simulink model "Aug_MPC_UnCon"  (R2021a)
settings: Solver=FixedStepDiscrete  StartTime=0.0  StopTime=10.0  FixedStep=h  RelTol=1e-3
values from neighbouring files (symbols this model uses):
  C = sys.C    [Initialize_MPC.m]    (also in Initialize_MPC_non.m; Values_Rev3.mat = [1 0 0 0 1 0 0 0 1 0 0 0 ... (18 elements, 3x6)])
  h = 0.01    [Main_Funwork4.m]
  K_Uncons = (matrices.R + matrices.Z'*matrices.Q*matrices.Z)^-1*matrices.Z'*matrices.Q    [Main_Funwork4.m]
  m = 3    [Main_Funwork4.m]
  Np = 43    [Main_Funwork4.m]
  r_p = zeros(m*Np,1)    [Initialize_MPC.m]    (also in Initialize_MPC_non.m = zeros(3*Np,1))
undefined symbols (not defined in the file or in its folder): constraints, DiscIntNeverNeededParam, int, matrices, x0
libraries: vrlib x2, simulink x1, aerolibanimutils x1, dspvision x1
settings Model: Creator=vicen  LastModifiedBy=vicen

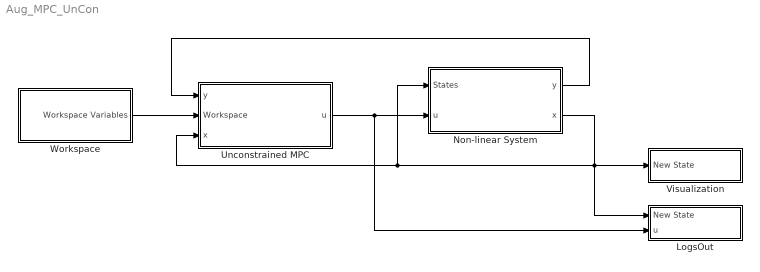
== system Aug_MPC_UnCon ==
  LogsOut : Subsystem
  Non-linear System : Subsystem
  Unconstrained MPC : Subsystem
  Visualization : Subsystem
  Workspace : Subsystem
  wires:
  Unconstrained MPC/1(u) -> LogsOut/2(u), Non-linear System/2(u)
  Non-linear System/1(y) -> Unconstrained MPC/1(y)
  Workspace/1(Workspace Variables) -> Unconstrained MPC/2(Workspace)
  Non-linear System/2(x) -> Visualization/1(New State), LogsOut/1(New State), Non-linear System/1(States), Unconstrained MPC/3(x)

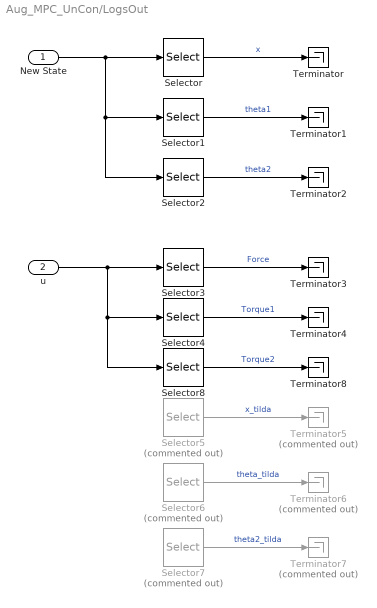
== system Aug_MPC_UnCon/LogsOut ==
  New State : Inport
  u : Inport  Port=2
  Selector : Selector  InputPortWidth=6  IndexOptions=Index vector (dialog)  Indices=1  OutputSizes=1
  Selector1 : Selector  InputPortWidth=6  IndexOptions=Index vector (dialog)  Indices=2  OutputSizes=1
  Selector2 : Selector  InputPortWidth=6  IndexOptions=Index vector (dialog)  Indices=3  OutputSizes=1
  Selector3 : Selector  InputPortWidth=3  IndexOptions=Index vector (dialog)  Indices=1  OutputSizes=1
  Selector4 : Selector  InputPortWidth=3  IndexOptions=Index vector (dialog)  Indices=2  OutputSizes=1
  Selector5 : Selector  Commented=on  InputPortWidth=6  IndexOptions=Index vector (dialog)  Indices=1  OutputSizes=1
  Selector6 : Selector  Commented=on  InputPortWidth=6  IndexOptions=Index vector (dialog)  Indices=2  OutputSizes=1
  Selector7 : Selector  Commented=on  InputPortWidth=6  IndexOptions=Index vector (dialog)  Indices=3  OutputSizes=1
  Selector8 : Selector  InputPortWidth=3  IndexOptions=Index vector (dialog)  Indices=3  OutputSizes=1
  Terminator{,1..4,8} (6 alike) : Terminator
  Terminator5 : Terminator  Commented=on
  Terminator6 : Terminator  Commented=on
  Terminator7 : Terminator  Commented=on
  wires:
  Selector/1 -> Terminator/1  "x"
  Selector1/1 -> Terminator1/1  "theta1"
  Selector2/1 -> Terminator2/1  "theta2"
  New State/1 -> Selector2/1, Selector1/1, Selector/1
  u/1 -> Selector8/1, Selector4/1, Selector3/1
  Selector4/1 -> Terminator4/1  "Torque1"
  Selector3/1 -> Terminator3/1  "Force"
  Selector5/1 -> Terminator5/1  "x_tilda"
  Selector6/1 -> Terminator6/1  "theta_tilda"
  Selector7/1 -> Terminator7/1  "theta2_tilda"
  Selector8/1 -> Terminator8/1  "Torque2"

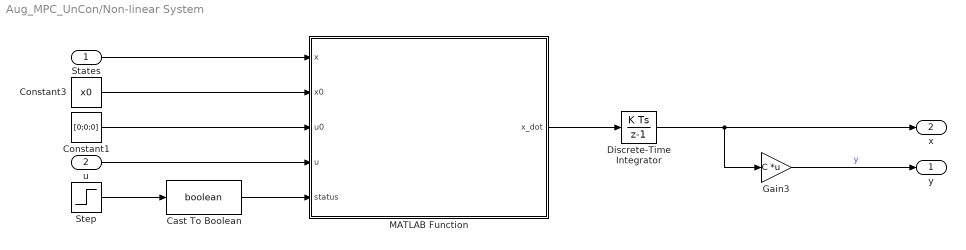
== system Aug_MPC_UnCon/Non-linear System ==
  States : Inport
  u : Inport  Port=2
  Cast To Boolean : DataTypeConversion  OutDataTypeStr=boolean
  Constant1 : Constant  Value=[0;0;0]  VectorParams1D=off
  Constant3 : Constant  Value=x0  VectorParams1D=off  OutDataTypeStr=Bus: State_bus
  Discrete-Time Integrator : DiscreteIntegrator  InitialCondition=[x0.x;x0.theta1;x0.theta2;x0.x_dot;x0.theta1_dot;x0.theta2_dot]  SampleTime=h  ICPrevOutput=DiscIntNeverNeededParam  ICPrevScaledInput=DiscIntNeverNeededParam
  Gain3 : Gain  Gain=C  Multiplication=Matrix(K*u)
  MATLAB Function : MATLAB Function  TreatAsAtomicUnit=on
  Step : Step  Time=h  SampleTime=0
  y : Outport
  x : Outport  Port=2
  wires:
  States/1 -> MATLAB Function/1(x)
  u/1 -> MATLAB Function/4(u)
  Step/1 -> Cast To Boolean/1
  Cast To Boolean/1 -> MATLAB Function/5(status)
  Gain3/1 -> y/1  "y"
  Discrete-Time Integrator/1 -> Gain3/1, x/1
  Constant3/1 -> MATLAB Function/2(x0)
  MATLAB Function/1(x_dot) -> Discrete-Time Integrator/1
  Constant1/1 -> MATLAB Function/3(u0)

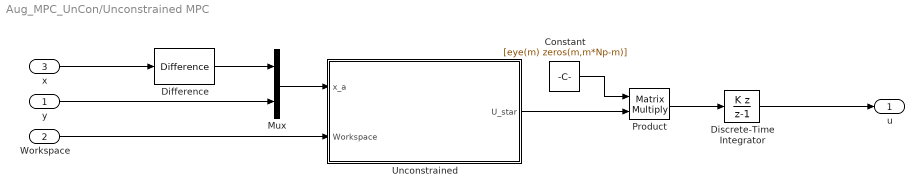
== system Aug_MPC_UnCon/Unconstrained MPC ==
  y : Inport
  Workspace : Inport  Port=2
  x : Inport  Port=3
  Constant : Constant  Value=[eye(m) zeros(m,m*Np-m)]  VectorParams1D=off
  Difference : simulink/Discrete/Difference  ICPrevInput=[x0.x;x0.theta1;x0.theta2;x0.x_dot;x0.theta1_dot;x0.theta2_dot]  OutMin=[]  OutMax=[]  OutDataType=fixdt(1, 16)  OutScaling=2^-10  DoSatur=off
  Discrete-Time Integrator : DiscreteIntegrator  IntegratorMethod=Accumulation: Backward Euler  InitialCondition=[0;0;0]  SampleTime=-1  ICPrevOutput=DiscIntNeverNeededParam  ICPrevScaledInput=DiscIntNeverNeededParam
  Mux : Mux  Inputs=2
  Product : Product  Multiplication=Matrix(*)
  Unconstrained : Subsystem
  u : Outport
  wires:
  Difference/1 -> Mux/1
  y/1 -> Mux/2
  Mux/1 -> Unconstrained/1(x_a)
  Workspace/1 -> Unconstrained/2(Workspace)
  Constant/1 -> Product/1
  Unconstrained/1(U_star) -> Product/2
  x/1 -> Difference/1
  Discrete-Time Integrator/1 -> u/1
  Product/1 -> Discrete-Time Integrator/1

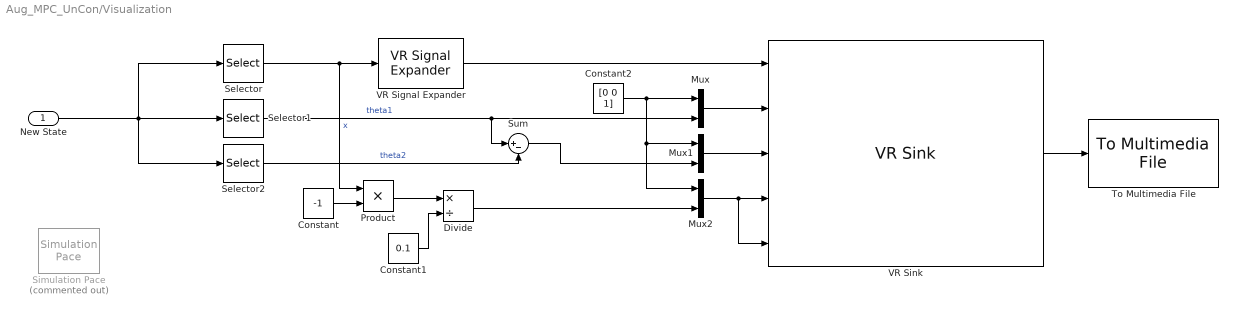
== system Aug_MPC_UnCon/Visualization ==
  New State : Inport
  Constant : Constant  Value=-1
  Constant1 : Constant  Value=0.1
  Constant2 : Constant  Value=[0 0 1]
  Divide : Product  Inputs=*/
  Mux : Mux  Inputs=2
  Mux1 : Mux  Inputs=2
  Mux2 : Mux  Inputs=2
  Product : Product
  Selector : Selector  InputPortWidth=6  IndexOptions=Index vector (dialog)  Indices=1  OutputSizes=1
  Selector1 : Selector  InputPortWidth=6  IndexOptions=Index vector (dialog)  Indices=2  OutputSizes=1
  Selector2 : Selector  InputPortWidth=6  IndexOptions=Index vector (dialog)  Indices=3  OutputSizes=1
  Simulation Pace : aerolibanimutils/Simulation Pace  Commented=on  SimulationPace=1  SleepMode=Auto  OutputPaceError=off  SampleTime=1/30
  Sum : Sum  Inputs=|+-
  To Multimedia File : dspvision/To Multimedia File  outputFilename=prob2.avi  streamSelection=Video only  videoCompressor=None (uncompressed)  audioCompressor=None (uncompressed)  imagePorts=One multidimensional signal  fileType=AVI  audioDatatype=Determine from input data type  fourcc=RGB  videoQuality=75  mj2000CompFactor=10
  VR Signal Expander : vrlib/VR Signal Expander  outwidth=3  outidx=[1]
  VR Sink : vrlib/VR Sink  InstantiateOnLoad=on  SampleTime=0.1  ViewEnable=on  RemoteChange=off  RemoteView=off  FieldsWritten=Cart.translation.3.1.1.double#Rotation1.rotation.4.1.1.double#Rotation2.rotation.4.1.1.double#Axis_Rotate.rotation.4.1.1.double#Axis_Rotate2.rotation.4.1.1.double  WorldFileName=Cart_Actual.WRL  AutoView=off  VideoDimensions=[1500 2000]  AllowVariableSize=off  FigureProperties="{'Position', 'Name', 'Viewpoint', 'CameraBound', 'CameraDirection', 'CameraPosition', 'CameraUpVector', 'ZoomFactor', 'Antialiasing', 'Headlight', 'Lighting', 'NavPanel', 'Sound', 'StatusBar', 'Stereo3D', 'Stereo3DCameraOffset', 'Stereo3DHIT', 'ToolBar', 'Textures', 'Transparency', 'Triad', 'Wireframe', 'NavZones', 'NavMode', 'NavSpeed', 'CaptureFileFormat', 'CaptureFileName', 'Record2DCompressMethod', 'Record2DCompressQuality', 'Record2D', 'Record2DFileName', 'Record2DFPS'; [1.2660000000000001e+02   9.4799999999999955e+01   8.0000000000000000e+02   6.0020000000000005e+02], '', '_untitled_1', 'on', [0.0000000000000000e+00   0.0000000000000000e+00  -1.0000000000000000e+00], [0.0000000000000000e+00   0.0000000000000000e+00   0.0000000000000000e+00], [0.0000000000000000e+00   1.0000000000000000e+00   0.0000000000000000e+00], [1.0000000000000000e+00], 'on', 'on', 'on', 'none', 'on', 'off', 'off', [1.0000000149011612e-01], [0.0000000000000000e+00], 'off', 'on', 'on', 'none', 'off', 'off', 'fly', 'normal', 'tif', '%f_anim_%n.tif', 'auto', [7.5000000000000000e+01], 'off', '***video***', 'auto'}"
  wires:
  New State/1 -> Selector/1, Selector2/1, Selector1/1
  Selector/1 -> VR Signal Expander/1, Product/1  "x"
  Selector1/1 -> Sum/1, Mux/2  "theta1"
  Product/1 -> Divide/1
  Constant/1 -> Product/2
  Constant1/1 -> Divide/2
  Constant2/1 -> Mux1/1, Mux2/1, Mux/1
  Selector2/1 -> Sum/2  "theta2"
  Divide/1 -> Mux2/2
  Sum/1 -> Mux1/2
  VR Signal Expander/1 -> VR Sink/1
  Mux/1 -> VR Sink/2
  Mux1/1 -> VR Sink/3
  Mux2/1 -> VR Sink/4, VR Sink/5
  VR Sink/1 -> To Multimedia File/1

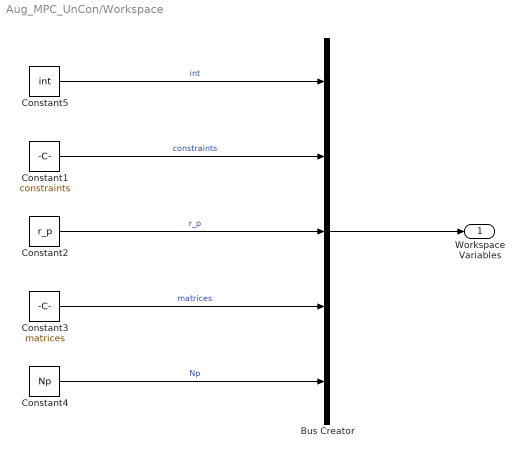
== system Aug_MPC_UnCon/Workspace ==
  Bus Creator : BusCreator  Inputs=5
  Constant1 : Constant  Value=constraints  VectorParams1D=off  OutDataTypeStr=Bus: Contraint_bus
  Constant2 : Constant  Value=r_p
  Constant3 : Constant  Value=matrices  VectorParams1D=off  OutDataTypeStr=Bus: Matrix_bus
  Constant4 : Constant  Value=Np  VectorParams1D=off
  Constant5 : Constant  Value=int  VectorParams1D=off  OutDataTypeStr=Bus: Initial_bus
  Workspace Variables : Outport
  wires:
  Bus Creator/1 -> Workspace Variables/1
  Constant1/1 -> Bus Creator/2  "constraints"
  Constant2/1 -> Bus Creator/3  "r_p"
  Constant3/1 -> Bus Creator/4  "matrices"
  Constant4/1 -> Bus Creator/5  "Np"
  Constant5/1 -> Bus Creator/1  "int"

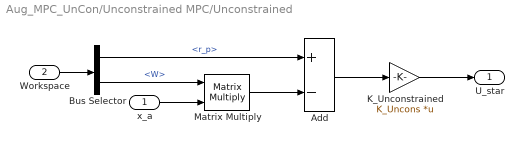
== system Aug_MPC_UnCon/Unconstrained MPC/Unconstrained ==
  x_a : Inport
  Workspace : Inport  Port=2
  Add : Sum  Inputs=+-
  Bus Selector : BusSelector  OutputSignals=r_p,matrices.W
  K_Unconstrained : Gain  Gain=K_Uncons  Multiplication=Matrix(K*u)
  Matrix Multiply : Product  Multiplication=Matrix(*)
  U_star : Outport
  wires:
  Workspace/1 -> Bus Selector/1
  Add/1 -> K_Unconstrained/1
  Matrix Multiply/1 -> Add/2
  K_Unconstrained/1 -> U_star/1
  Bus Selector/1 -> Add/1  "<r_p>"
  Bus Selector/2 -> Matrix Multiply/1  "<W>"
  x_a/1 -> Matrix Multiply/2

== matlab function Aug_MPC_UnCon/Non-linear System/MATLAB Function ==
  data: x input; x0 input; u0 input; u input; x_dot output; status input
function x_dot  = Nonlinear_Dynamics(x,x0,u0,u,status)
    if status == false
        x2 = x0.theta1;
        x3 = x0.theta2;
        x4 = x0.x_dot;
        x5 = x0.theta1_dot;
        x6 = x0.theta2_dot;
        u1 = u0(1);
        u2 = u0(2);
        u3 = u0(3);
    else
        x2 = x(2);
        x3 = x(3);
        x4 = x(4);
        x5 = x(5);
        x6 = x(6);
        u1 = u(1);
        u2 = u(2);
        u3 = u(3);
    end
    % Insert Equations
    x_dot = double([
                     x4;
                     x5;
                     x6;
                     -(420*u1 - (2943*sin(2*x2))/2 + 150*x5^2*sin(x2) + (135*x6^2*sin(x3))/2 - 180*u1*cos(2*x2 - 2*x3) + 400*u3*cos(2*x2 - x3) - 840*u2*cos(x2) + 840*u3*cos(x2) - 400*u3*cos(x3) + (135*x6^2*sin(2*x2 - x3))/2 + 360*u2*cos(x2 - 2*x3) - 360*u3*cos(x2 - 2*x3))/(30*(5*cos(2*x2) + 9*cos(2*x2 - 2*x3) - 26));
                     (22800*u3 - 22800*u2 - 26487*sin(x2 - 2*x3) - 91233*sin(x2) + 3600*u2*cos(2*x3) - 3600*u3*cos(2*x3) + 4725*x6^2*sin(x2 - x3) + 750*x5^2*sin(2*x2) - 4000*u3*cos(x2 + x3) + 4200*u1*cos(x2) + 1350*x5^2*sin(2*x2 - 2*x3) - 1800*u1*cos(x2 - 2*x3) + 13600*u3*cos(x2 - x3) + 675*x6^2*sin(x2 + x3))/(150*(5*cos(2*x2) + 9*cos(2*x2 - 2*x3) - 26));
                     -(2700*sin(x2 - x3)*x5^2 + 1215*sin(2*x2 - 2*x3)*x6^2 + 13600*u3 - 26487*sin(2*x2 - x3) + 26487*sin(x3) - 4000*u3*cos(2*x2) + 1800*u1*cos(2*x2 - x3) + 3600*u2*cos(x2 + x3) - 3600*u3*cos(x2 + x3) - 1800*u1*cos(x3) - 12240*u2*cos(x2 - x3) + 12240*u3*cos(x2 - x3))/(135*(5*cos(2*x2) + 9*cos(2*x2 - 2*x3) - 26))
                ]);
            
end
